simulink library "motor_loop_pump_and_fan_PWM_LVLibrary"  (R2020a)
settings: Solver=ode45  StartTime=0.0  StopTime=10.0  RelTol=1e-3  EnableMultiTasking=on
undefined symbols (not defined in the file): CR
libraries: simulink x4
settings Model: Creator=aldernl  LastModifiedBy=Harjot
settings DataIOCC: LimitDataPoints=on
settings OptimizationCC: LifeSpan=inf
settings DebuggingCC: AllowSymbolicDim=off  SFUnexpectedBacktrackingDiag=warning  SFNoUnconditionalDefaultTransitionDiag=warning  ArithmeticOperatorsInVariantConditions=warning
settings SFSimCC: SimUseLocalCustomCode=off  CustomCodeUndefinedFunction=UseInterfaceOnly
settings RTWCC: RTWUseLocalCustomCode=off
settings CodeAppCC: StateflowObjectComments=on
settings GRTTargetCC: TargetLangStandard=C89/C90 (ANSI)
settings ConfigComp: CovMetricSettings=dw  CovHtmlReporting=on  CovSaveCumulativeToWorkspaceVar=on  CovSaveSingleToWorkspaceVar=on  CovExternalEMLEnable=off

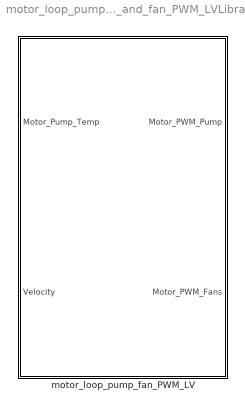
== system motor_loop_pump_and_fan_PWM_LVLibrary ==
  motor_loop_pump_fan_PWM_LV : Subsystem

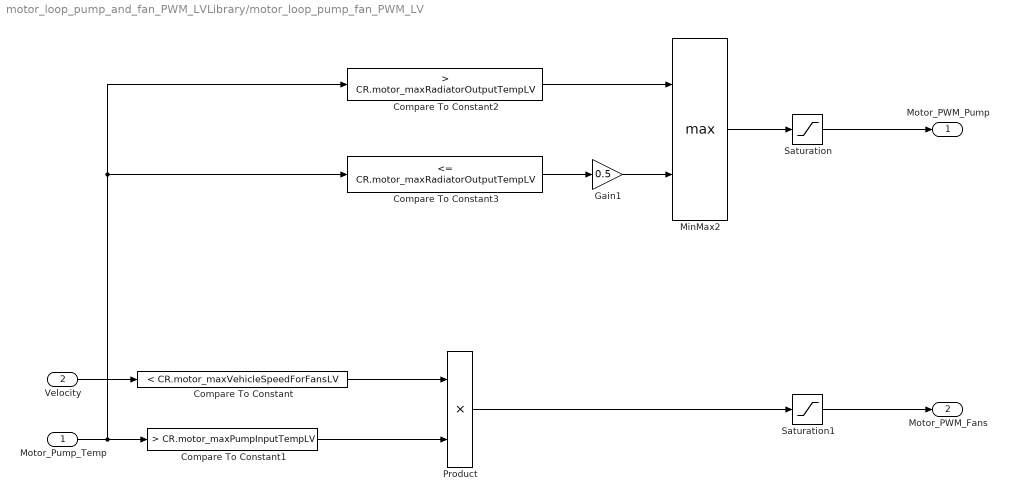
== system motor_loop_pump_and_fan_PWM_LVLibrary/motor_loop_pump_fan_PWM_LV ==
  Motor_Pump_Temp : Inport  OutDataTypeStr=double  PortDimensions=1
  Velocity : Inport  Port=2  OutDataTypeStr=double  PortDimensions=1
  Compare To Constant : simulink/Logic and Bit Operations/Compare To Constant  relop=<  const=CR.motor_maxVehicleSpeedForFansLV  OutDataTypeStr=boolean
  Compare To Constant1 : simulink/Logic and Bit Operations/Compare To Constant  relop=>  const=CR.motor_maxPumpInputTempLV  OutDataTypeStr=boolean
  Compare To Constant2 : simulink/Logic and Bit Operations/Compare To Constant  relop=>  const=CR.motor_maxRadiatorOutputTempLV  OutDataTypeStr=uint8
  Compare To Constant3 : simulink/Logic and Bit Operations/Compare To Constant  relop=<=  const=CR.motor_maxRadiatorOutputTempLV  OutDataTypeStr=uint8
  Gain1 : Gain  Gain=0.5
  MinMax2 : MinMax  Function=max  Inputs=2  OutDataTypeStr=double
  Product : Product  OutDataTypeStr=double
  Saturation : Saturate  UpperLimit=CR.motor_pump_saturation_LV  LowerLimit=0
  Saturation1 : Saturate  UpperLimit=CR.motor_fan_saturation_LV  LowerLimit=0
  Motor_PWM_Pump : Outport  OutDataTypeStr=double  PortDimensions=1  VectorParamsAs1DForOutWhenUnconnected=off
  Motor_PWM_Fans : Outport  Port=2  OutDataTypeStr=double  PortDimensions=1  VectorParamsAs1DForOutWhenUnconnected=off
  wires:
  Compare To Constant/1 -> Product/1
  Compare To Constant1/1 -> Product/2
  Velocity/1 -> Compare To Constant/1
  Motor_Pump_Temp/1 -> Compare To Constant1/1, Compare To Constant2/1, Compare To Constant3/1
  Compare To Constant3/1 -> Gain1/1
  Saturation/1 -> Motor_PWM_Pump/1
  MinMax2/1 -> Saturation/1
  Product/1 -> Saturation1/1
  Saturation1/1 -> Motor_PWM_Fans/1
  Compare To Constant2/1 -> MinMax2/1
  Gain1/1 -> MinMax2/2
